simulink model "Kinematics_Model"  (R2024a)
settings: Solver=VariableStepAuto  StartTime=0.0  StopTime=10.0  RelTol=1e-3
undefined symbols (not defined in the file): omega_b, p_b_i_0, q_0, v_b
settings Model: Creator=Usuario  LastModifiedBy=Usuario

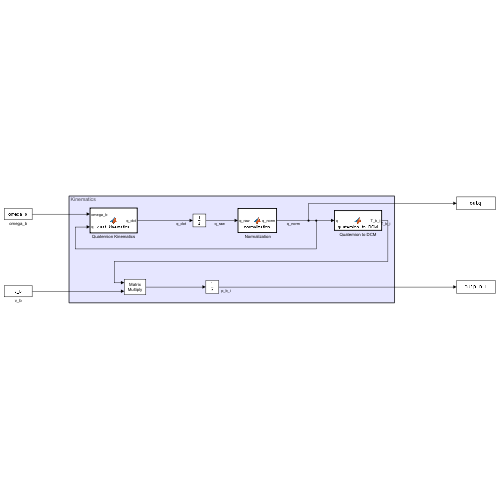
[thumbnail: Simulink's stored preview of the top-level diagram]
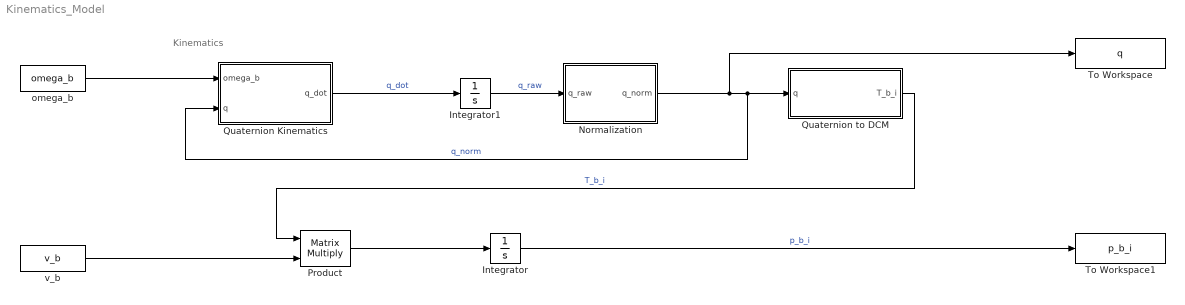
== system Kinematics_Model ==
  note: Kinematics
  " Normalization" : MATLAB Function  TreatAsAtomicUnit=on
  Integrator : Integrator  InitialCondition=p_b_i_0
  Integrator1 : Integrator  InitialCondition=q_0
  Product : Product  Multiplication=Matrix(*)
  Quaternion Kinematics : MATLAB Function  TreatAsAtomicUnit=on
  Quaternion to DCM : MATLAB Function  TreatAsAtomicUnit=on
  To Workspace : ToWorkspace  VariableName=q  SaveFormat=Timeseries  SampleTime=-1
  To Workspace1 : ToWorkspace  VariableName=p_b_i  SaveFormat=Timeseries  SampleTime=-1
  omega_b : Constant  Value=omega_b
  v_b : Constant  Value=v_b
  wires:
  omega_b/1 -> Quaternion Kinematics/1(omega_b)
  v_b/1 -> Product/2
  Quaternion to DCM/1(T_b_i) -> Product/1  "T_b_i"
  Product/1 -> Integrator/1
  Quaternion Kinematics/1(q_dot) -> Integrator1/1  "q_dot"
  Integrator/1 -> To Workspace1/1  "p_b_i"
  Integrator1/1 -> " Normalization"/1(q_raw)  "q_raw"
  " Normalization"/1(q_norm) -> To Workspace/1, Quaternion Kinematics/2(q), Quaternion to DCM/1(q)  "q_norm"

== matlab function Kinematics_Model/ Normalization ==
  data: q_raw input; q_norm output
function q_norm=normalization(q_raw)

q_norm=q_raw/norm(q_raw);

== matlab function Kinematics_Model/Quaternion Kinematics ==
  data: omega_b input; q_dot output; q input
function q_dot = quat_kinematics(omega_b,q)
%Quaternion kinematics. Requires that omega_b be a column vector. q must
%also be a column vector following the course's quaternion convention. 
eta=q(1);
epsilon=q(2:4);
epsilon_x=cross_matrix(epsilon);

q_dot=1/2*[-epsilon';epsilon_x+eta*eye(3,3)]*omega_b;
end

== matlab function Kinematics_Model/Quaternion to DCM ==
  data: q input; T_b_i output
function T_b_i=quaternion_to_DCM(q)
%My implementation of the quaternion to DCM transformation, to ensure
%consistency. It must return the active representation of the rotation
%between i and b, which will be the DCM from b to i. 
eta=q(1);
epsilon=q(2:4);
epsilon_x=cross_matrix(epsilon);

T_b_i=eye(3,3)+2*eta*epsilon_x+2*epsilon_x*epsilon_x;
end
